simulink model "experiment_simulation"  (R2023b)
settings: Solver=VariableStepAuto  StartTime=0.0  StopTime=27  RelTol=1e-3
InitFcn:
  | parameters
model workspace (MAT data in the model file):
  trajectory_a = [-1.52409846931 0.800900294758 0.522291166812 0.881049446282 0.615681685123 0.846225707965 -1.91228070877 1.70613035573 -0.416782684687 1.94182780206 0.715113366686 0.630917086666 ... (70 elements, 7x10)]
  trajectory_b = [1.63785922603 1.06519745333 0.917286904974 -0.0990593700309 -1.33458996905 1.44935684592 -1.71486047215 -1.76858838765 1.00521664875 1.43938283234 1.2212819449 -1.40157163353 ... (70 elements, 7x10)]
values from neighbouring files (symbols this model uses):
  m = length(U)-1    [bspline_findspan.m]
  param_robot = load_mu(param_robot, mu)    [parameters.m]
undefined symbols (not defined in the file or in its folder): par, param_initial_condition, param_sensor, X, Y, Z
libraries: nesl_utility x308, sm_lib x269, simulink_extras x1
(part 4 of 4)

== matlab function experiment_simulation/KUKA LBR iiwa reduced ==
  data: motion_enabled input; motor_enable input; tau_ext input; tau_m input; x input; dx output; param_robot parameter; tau_m_feedback output
function [dx,tau_m_feedback]   = fcn(motion_enabled,motor_enable, tau_ext, tau_m, x, param_robot)
  if(motion_enabled)
    q=x(1:7);           % generalized coordinates
    theta=x(8:14);      % motor angles
    q_p=x(15:21);       % time derivative of generalized coordinates
    theta_p=x(22:28);   % time derivative of motor angles
    
    motor_disable=(motor_enable~=1);
    tau_m(motor_disable)=0;
    
    M=inertia_matrix(q,param_robot);                    % inertia matrix
    C=coriolis_matrix(q,q_p,param_robot);               % coriolis matrix
    N=conservative_forces(q,q_p,theta,param_robot);     % conservative forces

    FS = diag([param_robot.FS1 param_robot.FS2 param_robot.FS3 param_robot.FS4 param_robot.FS5 param_robot.FS6 param_robot.FS7]);
    FV = diag([param_robot.FV1 param_robot.FV2 param_robot.FV3 param_robot.FV4 param_robot.FV5 param_robot.FV6 param_robot.FV7]);

    F = FS * sign(q_p) + FV * q_p;

    %disp("|M|=" + num2str(det(M)) + " - |C|=" + num2str(det(C)) + " - |g|"  + num2str(norm(N(1:7))));
    %sprintf("|M|= %0.5g - |C|= %0.5g - |g|= %0.5g - |theta-q| = %0.5g", det(M), det(C), norm(N(1:7)), norm(theta-q))

    dx=[q_p;...
      theta_p;...
      M\(tau_ext-C*q_p-N(1:7) - F);...
      param_robot.B\(tau_m-N(8:14))];
    
    dx(repmat(motor_disable,4,1))=0;
    tau_m_feedback=tau_m;
  else
    dx=zeros(size(x));
    tau_m_feedback=zeros(size(tau_m));
  end
end

== matlab function experiment_simulation/Filter ==
  data: x input; q output; q_p output
function [q,q_p] = fcn(x)
  q=x(1:7);
  q_p=x(15:21);
end

== matlab function experiment_simulation/Sensors/Sensor ==
  settings: sampleTime=param.T_a
  data: x input; theta output; param_robot parameter; tau output
function [theta,tau] = fcn(x,param_robot)
  q=x(1:7);
  theta=x(8:14);
  tau=param_robot.K*(theta-q);
end

== matlab function experiment_simulation/Motion Enable Logic/Motion Enable Logic ==
  data: motion_enable input; motion_enabled output; motion_disable input
function motion_enabled = fcn(motion_enable, motion_disable)
  persistent x_motion_enabled;

  if(isempty(x_motion_enabled))
      x_motion_enabled=0;
  end
  
  if(motion_disable)
    x_motion_enabled=0;
  elseif(motion_enable)
    x_motion_enabled=1;
  end
  
  motion_enabled=x_motion_enabled;
end

== matlab function experiment_simulation/External Force Generator ==
  data: channel input; F_ext output; value input; pulse input
function F_ext = fcn(channel,value,pulse)
  F_ext=zeros(6,1);
  if(pulse && channel>=1 && channel<=6)
    F_ext(channel)=value;
  end
end

== matlab function experiment_simulation/External Force Mapping ==
  data: x input; F_ext input; tau_ext output; param_robot parameter
function tau_ext = fcn(x, F_ext,param_robot)
  n=7;
  q=x(1:n);
  J=geo_jacobian_endeffector(q,param_robot);
  H=hom_transform_endeffector(q,param_robot);
  R_0_e=H(1:3,1:3);
  tau_ext=J'*[R_0_e,zeros(3);zeros(3),R_0_e]*F_ext;
end

== matlab function experiment_simulation/Visualisierung/Spur Endeffektor/MATLAB Function ==
  settings: updateMethod=DISCRETE  sampleTime=par.Ta
  data: q input; p1 output; p2 output; p3 output; p4 output; p5 output; p6 output; p7 output; p8 output; p9 output; p10 output; p11 output; p12 output; p13 output; p14 output; p15 output; p16 output; p17 output; p18 output; p19 output; p20 output; p21 output; p22 output; p23 output; p24 output; p25 output; p26 output; p27 output; p28 output; p29 output; p30 output; p31 output; p32 output; p33 output; p34 output; p35 output; p36 output; p37 output; p38 output; p39 output; p40 output; p41 output; p42 output; p43 output; p44 output; p45 output; p46 output; p47 output; p48 output; p49 output; p50 output; start input; delta input; p51 output; p52 output; p53 output; p54 output; p55 output; p56 output; p57 output; p58 output; p59 output; p60 output; p61 output; p62 output; p63 output; p64 output; p65 output; p66 output; p67 output; p68 output; p69 output; p70 output; p71 output; p72 output; p73 output; p74 output; p75 output; p76 output; p77 output; p78 output; p79 output; p80 output; p81 output; p82 output; p83 output; p84 output; p85 output; p86 output; p87 output; p88 output; p89 output; p90 output; p91 output; p92 output; p93 output; p94 output; p95 output; p96 output; p97 output; p98 output; p99 output; p100 output; param_robot parameter
function [p1,p2,p3,p4,p5,p6,p7,p8,p9,p10,p11,p12,p13,p14,p15,p16,p17,p18,p19,p20,p21,p22,p23,p24,p25,p26,p27,p28,p29,p30,p31,p32,p33,p34,p35,p36,p37,p38,p39,p40,p41,p42,p43,p44,p45,p46,p47,p48,p49,p50,p51,p52,p53,p54,p55,p56,p57,p58,p59,p60,p61,p62,p63,p64,p65,p66,p67,p68,p69,p70,p71,p72,p73,p74,p75,p76,p77,p78,p79,p80,p81,p82,p83,p84,p85,p86,p87,p88,p89,p90,p91,p92,p93,p94,p95,p96,p97,p98,p99,p100] = fcn(q, start, delta, param_robot)
persistent i t1 t2 t3 t4 t5 t6 t7 t8 t9 t10 t11 t12 t13 t14 t15 t16 t17 t18 t19 t20 t21 t22 t23 t24 t25 t26 t27 t28 t29 t30 t31 t32 t33 t34 t35 t36 t37 t38 t39 t40 t41 t42 t43 t44 t45 t46 t47 t48 t49 t50 t51 t52 t53 t54 t55 t56 t57 t58 t59 t60 t61 t62 t63 t64 t65 t66 t67 t68 t69 t70 t71 t72 t73 t74 t75 t76 t77 t78 t79 t80 t81 t82 t83 t84 t85 t86 t87 t88 t89 t90 t91 t92 t93 t94 t95 t96 t97 t98 t99 t100
H=hom_transform_endeffector(q,param_robot);
if isempty(t1)
    i = 1;
    t1 = H(1:3,4);
    t2 = t1;
    t3 = t1;
    t4 = t1;
    t5 = t1;
    t6 = t1;
    t7 = t1;
    t8 = t1;
    t9 = t1;
    t10 = t1;
    t11 = t1;
    t12 = t1;
    t13 = t1;
    t14 = t1;
    t15 = t1;
    t16 = t1;
    t17 = t1;
    t18 = t1;
    t19 = t1;
    t20 = t1;
    t21 = t1;
    t22 = t1;
    t23 = t1;
    t24 = t1;
    t25 = t1;
    t26 = t1;
    t27 = t1;
    t28 = t1;
    t29 = t1;
    t30 = t1;
    t31 = t1;
    t32 = t1;
    t33 = t1;
    t34 = t1;
    t35 = t1;
    t36 = t1;
    t37 = t1;
    t38 = t1;
    t39 = t1;
    t40 = t1;
    t41 = t1;
    t42 = t1;
    t43 = t1;
    t44 = t1;
    t45 = t1;
    t46 = t1;
    t47 = t1;
    t48 = t1;
    t49 = t1;
    t50 = t1;
    t51 = t1;
    t52 = t1;
    t53 = t1;
    t54 = t1;
    t55 = t1;
    t56 = t1;
    t57 = t1;
    t58 = t1;
    t59 = t1;
    t60 = t1;
    t61 = t1;
    t62 = t1;
    t63 = t1;
    t64 = t1;
    t65 = t1;
    t66 = t1;
    t67 = t1;
    t68 = t1;
    t69 = t1;
    t70 = t1;
    t71 = t1;
    t72 = t1;
    t73 = t1;
    t74 = t1;
    t75 = t1;
    t76 = t1;
    t77 = t1;
    t78 = t1;
    t79 = t1;
    t80 = t1;
    t81 = t1;
    t82 = t1;
    t83 = t1;
    t84 = t1;
    t85 = t1;
    t86 = t1;
    t87 = t1;
    t88 = t1;
    t89 = t1;
    t90 = t1;
    t91 = t1;
    t92 = t1;
    t93 = t1;
    t94 = t1;
    t95 = t1;
    t96 = t1;
    t97 = t1;
    t98 = t1;
    t99 = t1;
    t100 = t1;
    
end

switch i
    case start
        t1 = H(1:3,4);
    case start+delta*1
        t2 = H(1:3,4);
    case start+delta*2
        t3 = H(1:3,4);
    case start+delta*3
        t4 = H(1:3,4);
    case start+delta*4
        t5 = H(1:3,4);
    case start+delta*5
        t6 = H(1:3,4);
    case start+delta*6
        t7 = H(1:3,4);
    case start+delta*7
        t8 = H(1:3,4);
    case start+delta*8
        t9 = H(1:3,4);
    case start+delta*9
        t10 = H(1:3,4);
    case start+delta*10
        t11 = H(1:3,4);
    case start+delta*11
        t12 = H(1:3,4);
    case start+delta*12
        t13 = H(1:3,4);
    case start+delta*13
        t14 = H(1:3,4);
    case start+delta*14
        t15 = H(1:3,4);
    case start+delta*15
        t16 = H(1:3,4);
    case start+delta*16
        t17 = H(1:3,4);
    case start+delta*17
        t18 = H(1:3,4);
    case start+delta*18
        t19 = H(1:3,4);
    case start+delta*19
        t20 = H(1:3,4);
    case start+delta*20
        t21 = H(1:3,4);
    case start+delta*21
        t22 = H(1:3,4);
    case start+delta*22
        t23 = H(1:3,4);
    case start+delta*23
        t24 = H(1:3,4);
    case start+delta*24
        t25 = H(1:3,4);
    case start+delta*25
        t26 = H(1:3,4);
    case start+delta*26
        t27 = H(1:3,4);
    case start+delta*27
        t28 = H(1:3,4);
    case start+delta*28
        t29 = H(1:3,4);
    case start+delta*29
        t30 = H(1:3,4);
    case start+delta*30
        t31 = H(1:3,4);
    case start+delta*31
        t32 = H(1:3,4);
    case start+delta*32
        t33 = H(1:3,4);
    case start+delta*33
        t34 = H(1:3,4);
    case start+delta*34
        t35 = H(1:3,4);
    case start+delta*35
        t36 = H(1:3,4);
    case start+delta*36
        t37 = H(1:3,4);
    case start+delta*37
        t38 = H(1:3,4);
    case start+delta*38
        t39 = H(1:3,4);
    case start+delta*39
        t40 = H(1:3,4);
    case start+delta*40
        t41 = H(1:3,4);
    case start+delta*41
        t42 = H(1:3,4);
    case start+delta*42
        t43 = H(1:3,4);
    case start+delta*43
        t44 = H(1:3,4);
    case start+delta*44
        t45 = H(1:3,4);
    case start+delta*45
        t46 = H(1:3,4);
    case start+delta*46
        t47 = H(1:3,4);
    case start+delta*47
        t48 = H(1:3,4);
    case start+delta*48
        t49 = H(1:3,4);
    case start+delta*49
        t50 = H(1:3,4);
    case start+delta*50
        t51 = H(1:3,4);
    case start+delta*51
        t52 = H(1:3,4);
    case start+delta*52
        t53 = H(1:3,4);
    case start+delta*53
        t54 = H(1:3,4);
    case start+delta*54
        t55 = H(1:3,4);
    case start+delta*55
        t56 = H(1:3,4);
    case start+delta*56
        t57 = H(1:3,4);
    case start+delta*57
        t58 = H(1:3,4);
    case start+delta*58
        t59 = H(1:3,4);
    case start+delta*59
        t60 = H(1:3,4);
    case start+delta*60
        t61 = H(1:3,4);
    case start+delta*61
        t62 = H(1:3,4);
    case start+delta*62
        t63 = H(1:3,4);
    case start+delta*63
        t64 = H(1:3,4);
    case start+delta*64
        t65 = H(1:3,4);
    case start+delta*65
        t66 = H(1:3,4);
    case start+delta*66
        t67 = H(1:3,4);
    case start+delta*67
        t68 = H(1:3,4);
    case start+delta*68
        t69 = H(1:3,4);
    case start+delta*69
        t70 = H(1:3,4);
    case start+delta*70
        t71 = H(1:3,4);
    case start+delta*71
        t72 = H(1:3,4);
    case start+delta*72
        t73 = H(1:3,4);
    case start+delta*73
        t74 = H(1:3,4);
    case start+delta*74
        t75 = H(1:3,4);
    case start+delta*75
        t76 = H(1:3,4);
    case start+delta*76
        t77 = H(1:3,4);
    case start+delta*77
        t78 = H(1:3,4);
    case start+delta*78
        t79 = H(1:3,4);
    case start+delta*79
        t80 = H(1:3,4);
    case start+delta*80
        t81 = H(1:3,4);
    case start+delta*81
        t82 = H(1:3,4);
    case start+delta*82
        t83 = H(1:3,4);
    case start+delta*83
        t84 = H(1:3,4);
    case start+delta*84
        t85 = H(1:3,4);
    case start+delta*85
        t86 = H(1:3,4);
    case start+delta*86
        t87 = H(1:3,4);
    case start+delta*87
        t88 = H(1:3,4);
    case start+delta*88
        t89 = H(1:3,4);
    case start+delta*89
        t90 = H(1:3,4);
    case start+delta*90
        t91 = H(1:3,4);
    case start+delta*91
        t92 = H(1:3,4);
    case start+delta*92
        t93 = H(1:3,4);
    case start+delta*93
        t94 = H(1:3,4);
    case start+delta*94
        t95 = H(1:3,4);
    case start+delta*95
        t96 = H(1:3,4);
    case start+delta*96
        t97 = H(1:3,4);
    case start+delta*97
        t98 = H(1:3,4);
    case start+delta*98
        t99 = H(1:3,4);
    case start+delta*99
        t100 = H(1:3,4);
end

i = i+1;
p1 = t1;
p2 = t2;
p3 = t3;
p4 = t4;
p5 = t5;
p6 = t6;
p7 = t7;
p8 = t8;
p9 = t9;
p10 = t10;
p11 = t11;
p12 = t12;
p13 = t13;
p14 = t14;
p15 = t15;
p16 = t16;
p17 = t17;
p18 = t18;
p19 = t19;
p20 = t20;
p21 = t21;
p22 = t22;
p23 = t23;
p24 = t24;
p25 = t25;
p26 = t26;
p27 = t27;
p28 = t28;
p29 = t29;
p30 = t30;
p31 = t31;
p32 = t32;
p33 = t33;
p34 = t34;
p35 = t35;
p36 = t36;
p37 = t37;
p38 = t38;
p39 = t39;
p40 = t40;
p41 = t41;
p42 = t42;
p43 = t43;
p44 = t44;
p45 = t45;
p46 = t46;
p47 = t47;
p48 = t48;
p49 = t49;
p50 = t50;
p51 = t51;
p52 = t52;
p53 = t53;
p54 = t54;
p55 = t55;
p56 = t56;
p57 = t57;
p58 = t58;
p59 = t59;
p60 = t60;
p61 = t61;
p62 = t62;
p63 = t63;
p64 = t64;
p65 = t65;
p66 = t66;
p67 = t67;
p68 = t68;
p69 = t69;
p70 = t70;
p71 = t71;
p72 = t72;
p73 = t73;
p74 = t74;
p75 = t75;
p76 = t76;
p77 = t77;
p78 = t78;
p79 = t79;
p80 = t80;
p81 = t81;
p82 = t82;
p83 = t83;
p84 = t84;
p85 = t85;
p86 = t86;
p87 = t87;
p88 = t88;
p89 = t89;
p90 = t90;
p91 = t91;
p92 = t92;
p93 = t93;
p94 = t94;
p95 = t95;
p96 = t96;
p97 = t97;
p98 = t98;
p99 = t99;
p100 = t100;
